simulink model "Trans_matlab2017"  (R2018b)
settings: Solver=VariableStepAuto  StartTime=0.0  StopTime=0.1  RelTol=1e-3
undefined symbols (not defined in the file): dUk_z, fn, L_load, R_load, Rpu, Ru_z, Sn_trans, U1, U2, Xpu, Xu_z
libraries: powerlib x14, powerlib_meascontrol x6
settings Model: Creator=Александр  LastModifiedBy=VID Company
settings DataIOCC: ReturnWorkspaceOutputs=on
settings DebuggingCC: UnconnectedInputMsg=none  UnconnectedOutputMsg=none  UnconnectedLineMsg=none
settings ModelReferenceCC: EnableRefExpFcnMdlSchedulingChecks=off
settings RTWCC: Description=Generic Real-Time Target

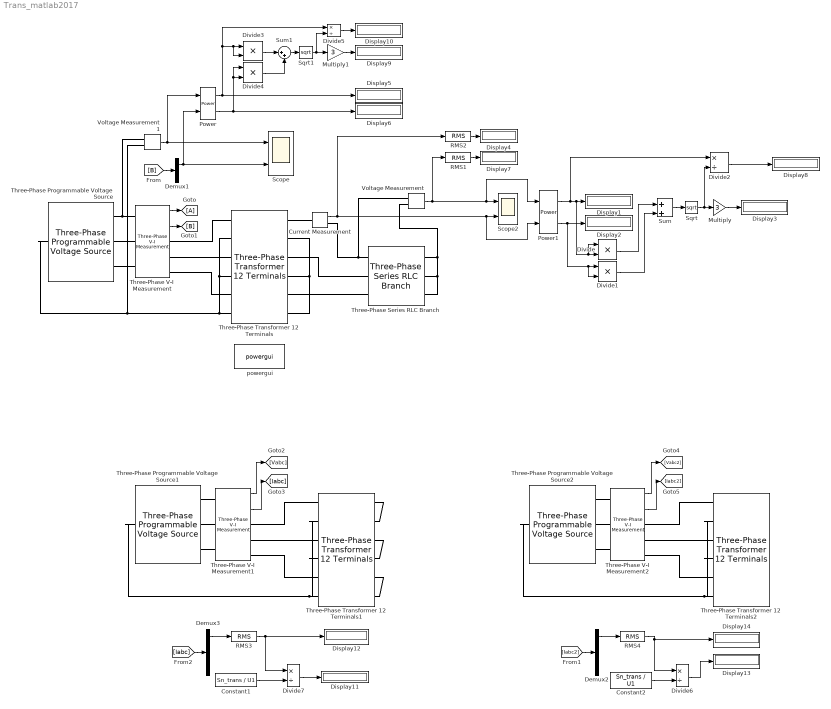
== system Trans_matlab2017 ==
  Constant1 : Constant  Value=Sn_trans / U1
  Constant2 : Constant  Value=Sn_trans / U1
  Current Measurement : powerlib/Measurements/Current Measurement  PhasorSimulation=off  OutputType=Complex  PSBequivalent=0
  Demux1 : Demux  Outputs=3
  Demux2 : Demux  Outputs=3
  Demux3 : Demux  Outputs=3
  Display{1..14} (14 alike) : Display
  Divide{,1,3..4} (4 alike) : Product  Inputs=**
  Divide{2,5..7} (4 alike) : Product  Inputs=*/
  Multiply : Gain  Gain=3
  Multiply1 : Gain  Gain=3
  Power : powerlib_meascontrol/Measurements/Power  Freq=fn  Vinit=[1, 0]  Iinit=[1, 0]  Ts=0
      settings: SourceProductName=Simscape Power Systems
  Power1 : powerlib_meascontrol/Measurements/Power  Freq=fn  Vinit=[1, 0]  Iinit=[1, 0]  Ts=0
      settings: SourceProductName=Simscape Power Systems
  RMS{1..4} (4 alike) : powerlib_meascontrol/Measurements/RMS  TrueRMS=on  Freq=fn  RMSInit=1  Ts=0
  Scope : Scope  NumInputPorts=2
  Scope2 : Scope  NumInputPorts=2
  Sqrt : Sqrt  SaturateOnIntegerOverflow=on
  Sqrt1 : Sqrt  SaturateOnIntegerOverflow=on
  Sum : Sum  Inputs=|++
  Sum1 : Sum  Inputs=|++
  Three-Phase Programmable Voltage Source : powerlib/Electrical Sources/Three-Phase Programmable Voltage Source  PositiveSequence="[U1*sqrt(3)  0 fn]"  VariationEntity=None  VariationType=Table of time-amplitude pairs  VariationTypeAlt=Step  VariationStep=0.5  VariationRate=10  VariationMagnitude=0.3  VariationFrequency=2  VariationTiming=[1 2]  VariationPhaseA=off  Amplitudes=[1 0.8 1.2 1.0]  TimeValues=[0 0.1 0.15 0.2]  HarmonicGeneration=off  HarmonicA=[3 0.2 -25 0]  HarmonicB=[2 0.15 35 2]  Timing="[0.05  3]"  BusType=swing  Pref=0  Qref=0  Qmin=-inf  Qmax=inf
  Three-Phase Programmable Voltage Source1 : powerlib/Electrical Sources/Three-Phase Programmable Voltage Source  PositiveSequence="[(dUk_z/100)*U1*sqrt(3)  0 fn]"  VariationEntity=None  VariationType=Table of time-amplitude pairs  VariationTypeAlt=Step  VariationStep=0.5  VariationRate=10  VariationMagnitude=0.3  VariationFrequency=2  VariationTiming=[1 2]  VariationPhaseA=off  Amplitudes=[1 0.8 1.2 1.0]  TimeValues=[0 0.1 0.15 0.2]  HarmonicGeneration=off  HarmonicA=[3 0.2 -25 0]  HarmonicB=[2 0.15 35 2]  Timing="[0.05  3]"  BusType=swing  Pref=0  Qref=0  Qmin=-inf  Qmax=inf
  Three-Phase Programmable Voltage Source2 : powerlib/Electrical Sources/Three-Phase Programmable Voltage Source  PositiveSequence=[U1*sqrt(3) 0 fn]  VariationEntity=None  VariationType=Table of time-amplitude pairs  VariationTypeAlt=Step  VariationStep=0.5  VariationRate=10  VariationMagnitude=0.3  VariationFrequency=2  VariationTiming=[1 2]  VariationPhaseA=off  Amplitudes=[1 0.8 1.2 1.0]  TimeValues=[0 0.1 0.15 0.2]  HarmonicGeneration=off  HarmonicA=[3 0.2 -25 0]  HarmonicB=[2 0.15 35 2]  Timing="[0.05  3]"  BusType=swing  Pref=0  Qref=0  Qmin=-inf  Qmax=inf
  Three-Phase Series RLC Branch : powerlib/Elements/Three-Phase Series RLC Branch  LConnTagsString=A|B|C  RConnTagsString=A|B|C  BranchType=RL  Resistance=R_load*0.93  Inductance=L_load  Capacitance=1e-6  Measurements=None
  Three-Phase V-I Measurement : powerlib/Measurements/Three-Phase V-I Measurement  VoltageMeasurement=phase-to-phase  SetLabelV=off  LabelV=Vabc  Vpu=off  VpuLL=off  CurrentMeasurement=yes  SetLabelI=off  LabelI=Iabc  Ipu=off  Pbase=100e6  Vbase=500e3  OutputType=Complex  PhasorSimulation=off  PSBequivalent=0
  Three-Phase V-I Measurement1 : powerlib/Measurements/Three-Phase V-I Measurement  VoltageMeasurement=phase-to-phase  SetLabelV=off  LabelV=Vabc  Vpu=off  VpuLL=off  CurrentMeasurement=yes  SetLabelI=off  LabelI=Iabc  Ipu=off  Pbase=100e6  Vbase=500e3  OutputType=Complex  PhasorSimulation=off  PSBequivalent=0
  Three-Phase V-I Measurement2 : powerlib/Measurements/Three-Phase V-I Measurement  VoltageMeasurement=phase-to-phase  SetLabelV=off  LabelV=Vabc  Vpu=off  VpuLL=off  CurrentMeasurement=yes  SetLabelI=off  LabelI=Iabc  Ipu=off  Pbase=100e6  Vbase=500e3  OutputType=Complex  PhasorSimulation=off  PSBequivalent=0
  Three-Phase Transformer 12 Terminals : powerlib/Elements/Three-Phase Transformer 12 Terminals  RatedPower=[ Sn_trans *3 fn ]  Winding1="[ U1 Rpu  Xpu]"  Winding2=[ U2 Rpu Xpu]  RmXm=[ Ru_z Xu_z]
      settings: SourceProductName=Simscape Power Systems  SourceProductBaseCode=PS
  Three-Phase Transformer 12 Terminals1 : powerlib/Elements/Three-Phase Transformer 12 Terminals  RatedPower=[ Sn_trans *3 fn ]  Winding1="[ U1 Rpu  Xpu]"  Winding2=[ U2 Rpu Xpu]  RmXm=[Ru_z Xu_z]
      settings: SourceProductName=Simscape Power Systems  SourceProductBaseCode=PS
  Three-Phase Transformer 12 Terminals2 : powerlib/Elements/Three-Phase Transformer 12 Terminals  RatedPower=[ Sn_trans *3 fn ]  Winding1="[ U1 Rpu  Xpu]"  Winding2=[ U2 Rpu Xpu]  RmXm=[Ru_z Xu_z]
      settings: SourceProductName=Simscape Power Systems  SourceProductBaseCode=PS
  Voltage Measurement : powerlib/Measurements/Voltage Measurement  PhasorSimulation=off  OutputType=Complex  PSBequivalent=0
  Voltage Measurement1 : powerlib/Measurements/Voltage Measurement  PhasorSimulation=off  OutputType=Complex  PSBequivalent=0
  powergui : powerlib/powergui  Priority=1  SimulationMode=Discrete  SampleTime=1e-6  frequency=60  Iterations=50  frequencyindice=400  Pbase=100e6  ErrMax=1e-4  UnitsV=kV  UnitsW=MW  buscounter=0  FunctionMessages=off  echomessages=off  EnableUseOfTLC=off  CurrentSourceSwitches=off  DisableSnubberDevices=off  DisableRonSwitches=off  DisableVfSwitches=off  DisplayEquations=off  SolverType=Tustin/Backward Euler (TBE)  Interpol=off  ExternalGateDelay=off  methode=off  Ts=100  x0status=blocks  SPID=on  SwTol=0  HookPort=off  RestoreLinks=warning  ResistiveCurrentMeasurement=off  Frange=[0:2:500]  Ylog=off  Xlog=on  ShowGrid=off  save=off  variable=ZData  structure=0  ZoomFFT=off  StartTime=0.0  cycles=1  DisplayStyle=1  fundamental=60  FreqAxis=off  MaxFrequency=1000  frequencyindicesteady=1  RmsSteady=1  display=off
  wires:
  Three-Phase V-I Measurement/1 -> [A]
  Three-Phase V-I Measurement/2 -> [B]
  Voltage Measurement1/1 -> Scope/1, Power/1
  Demux1/1 -> Scope/2, Power/2
  Power/1 -> Divide3/2, Divide3/1, Divide5/1, Display5/1
  [B] -> Demux1/1
  Power1/2 -> Display2/1, Divide1/2, Divide1/1
  Power1/1 -> Divide2/1, Divide/1, Divide/2, Display1/1
  Voltage Measurement/1 -> Power1/1, Scope2/1, RMS1/1
  Current Measurement/1 -> Power1/2, Scope2/2, RMS2/1
  Divide/1 -> Sum/1
  Divide1/1 -> Sum/2
  Multiply/1 -> Display3/1
  Sum/1 -> Sqrt/1
  Sqrt/1 -> Divide2/2, Multiply/1
  RMS1/1 -> Display7/1
  RMS2/1 -> Display4/1
  Divide2/1 -> Display8/1
  Power/2 -> Display6/1, Divide4/1, Divide4/2
  Sum1/1 -> Sqrt1/1
  Multiply1/1 -> Display9/1
  Sqrt1/1 -> Multiply1/1, Divide5/2
  Divide3/1 -> Sum1/1
  Divide4/1 -> Sum1/2
  Divide5/1 -> Display10/1
  Three-Phase V-I Measurement1/1 -> [Vabc]
  Three-Phase V-I Measurement1/2 -> [Iabc]
  [Iabc] -> Demux3/1
  Demux3/1 -> RMS3/1
  Three-Phase V-I Measurement2/2 -> [Iabc2]
  Three-Phase V-I Measurement2/1 -> [Vabc2]
  Constant1/1 -> Divide7/2
  Divide7/1 -> Display11/1
  RMS3/1 -> Divide7/1, Display12/1
  Constant2/1 -> Divide6/2
  Divide6/1 -> Display13/1
  Demux2/1 -> RMS4/1
  RMS4/1 -> Divide6/1, Display14/1
  [Iabc2] -> Demux2/1
  connections:
  Three-Phase V-I Measurement/LConn1 -- Voltage Measurement1/LConn1 -- Three-Phase Programmable Voltage Source/RConn1
  Three-Phase Programmable Voltage Source/RConn2 -- Three-Phase V-I Measurement/LConn2
  Three-Phase Programmable Voltage Source/RConn3 -- Three-Phase V-I Measurement/LConn3
  Three-Phase Series RLC Branch/LConn3 -- Three-Phase Transformer 12 Terminals/RConn5
  Current Measurement/RConn1 -- Voltage Measurement/LConn1 -- Three-Phase Series RLC Branch/LConn1
  Three-Phase Series RLC Branch/RConn1 -- Voltage Measurement/LConn2 -- Three-Phase Series RLC Branch/RConn3 -- Three-Phase Series RLC Branch/RConn2
  Three-Phase V-I Measurement/RConn1 -- Three-Phase Transformer 12 Terminals/LConn1
  Three-Phase V-I Measurement/RConn2 -- Three-Phase Transformer 12 Terminals/LConn3
  Three-Phase V-I Measurement/RConn3 -- Three-Phase Transformer 12 Terminals/LConn5
  Three-Phase Programmable Voltage Source/LConn1 -- Voltage Measurement1/LConn2 -- Three-Phase Transformer 12 Terminals/LConn2 -- Three-Phase Transformer 12 Terminals/LConn4 -- Three-Phase Transformer 12 Terminals/LConn6
  Three-Phase Transformer 12 Terminals/RConn1 -- Current Measurement/LConn1
  Three-Phase Transformer 12 Terminals/RConn3 -- Three-Phase Series RLC Branch/LConn2
  Three-Phase Transformer 12 Terminals/RConn2 -- Three-Phase Transformer 12 Terminals/RConn6 -- Three-Phase Transformer 12 Terminals/RConn4
  Three-Phase Transformer 12 Terminals1/LConn6 -- Three-Phase Programmable Voltage Source1/LConn1 -- Three-Phase Transformer 12 Terminals1/LConn4 -- Three-Phase Transformer 12 Terminals1/LConn2
  Three-Phase V-I Measurement1/LConn1 -- Three-Phase Programmable Voltage Source1/RConn1
  Three-Phase V-I Measurement1/RConn2 -- Three-Phase Transformer 12 Terminals1/LConn3
  Three-Phase V-I Measurement1/RConn1 -- Three-Phase Transformer 12 Terminals1/LConn1
  Three-Phase Programmable Voltage Source1/RConn2 -- Three-Phase V-I Measurement1/LConn2
  Three-Phase Programmable Voltage Source1/RConn3 -- Three-Phase V-I Measurement1/LConn3
  Three-Phase V-I Measurement1/RConn3 -- Three-Phase Transformer 12 Terminals1/LConn5
  Three-Phase Transformer 12 Terminals1/RConn1 -- Three-Phase Transformer 12 Terminals1/RConn2
  Three-Phase Transformer 12 Terminals1/RConn3 -- Three-Phase Transformer 12 Terminals1/RConn4
  Three-Phase Transformer 12 Terminals1/RConn5 -- Three-Phase Transformer 12 Terminals1/RConn6
  Three-Phase Transformer 12 Terminals2/LConn6 -- Three-Phase Programmable Voltage Source2/LConn1 -- Three-Phase Transformer 12 Terminals2/LConn4 -- Three-Phase Transformer 12 Terminals2/LConn2
  Three-Phase V-I Measurement2/RConn3 -- Three-Phase Transformer 12 Terminals2/LConn5
  Three-Phase Programmable Voltage Source2/RConn2 -- Three-Phase V-I Measurement2/LConn2
  Three-Phase V-I Measurement2/RConn1 -- Three-Phase Transformer 12 Terminals2/LConn1
  Three-Phase V-I Measurement2/RConn2 -- Three-Phase Transformer 12 Terminals2/LConn3
  Three-Phase Programmable Voltage Source2/RConn3 -- Three-Phase V-I Measurement2/LConn3
  Three-Phase V-I Measurement2/LConn1 -- Three-Phase Programmable Voltage Source2/RConn1
